simulink library "cstblocks"  (Simulink 7.4)
settings: Solver=ode45  SolverMode=SingleTasking  StartTime=0.0  StopTime=10.0  RelTol=1e-3
values from neighbouring files (symbols this model uses):
  D = diag(D)    [care.m]    (also in delayss.m = getPrivateData(sys); gcare.m = []; gdare.m = [])
libraries: cstextras x3
settings Model: RequirementInfo=9  ForwardingTableString=||__slOldName__||cstblocks/Output Point||__slNewName__||slctrlobsolete/Output Point||__slOldName__||cstblocks/Input Point||__slNewName__||slctrlobsolete/Input Point  Creator=greg  LastModifiedBy=pascal

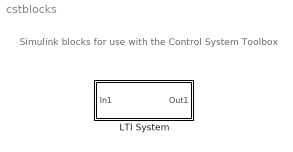
== system cstblocks ==
  note: Simulink blocks for use with the
      | Control System Toolbox
  LTI System : Subsystem  BlockChoice=CSS  mask(LTI Block){sys=tf(1,[1 1]), IC=[]}
      mask prompts: sys "LTI system variable"; IC "Initial states (state-space only)"
      mask help:
      | The LTI System block accepts both continuous and discrete LTI models as defined in the Control System Toolbox. Transfer function, state-space, and zero-pole-gain formats are all supported in this block.
      |
      | Note: Initial states are only meaningful for state-space systems.
      mask init:
      | try
      |    % read data to initialize mask variables
      |    [D,Ts,Tdi,Tdo,Tdio,x0,sysname]=...
      |       ltimask('Initialize',gcb,sys,IC);
      |    % update contents
      |    model = bdroot;
      |    df = get_param(model,'dirty');
      |    ltimask('UpdateDiagram',gcb,D,Ts,Tdio);
      |    try      
      |       % Attempt to modify locked library -> error
      |       % Makes block show ??? when loading CSTBLOCKS
      |       % for the first time
      |       set_param(model,'dirty',df)
      |    end
      | catch ME
      |    sys = [];  IC = [];   sysname = '???';
      |    throw(ME)
      | end
      mask Help:
      | The LTI System block accepts any of the three standard LTI models described in the Control System Toolbox: transfer function, zero/pole/gain, or state space. Internally, LTI models will be converted to their state space equivalent for evaluation.
      | <p>
      | In the editable text box labeled <b>LTI System Variable</b>, enter a valid LTI model.
      | <p>
      | In the editable text box labeled <b>Initial States</b> enter the initial state vector.  Initial states are only valid for state-space systems.
      | <p>
      | See also TF, ZPK, SS, LTIMODELS.
      mask CallbackString: ltimask('MaskLTICallback',gcb);|
      mask Display: disp(sysname)

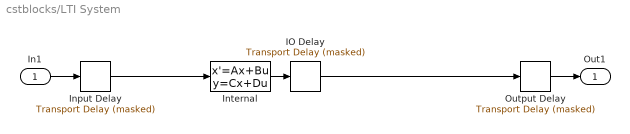
== system cstblocks/LTI System ==
  In1 : Inport  OutDataType=sfix(16)  OutScaling=2^0
  IO Delay : cstextras/Transport Delay (masked)  SystemSampleTime=-1  Td=Tdio  u0=0  bufsize=1024
  Input Delay : cstextras/Transport Delay (masked)  SystemSampleTime=-1  Td=Tdi  u0=0  bufsize=1024
  Internal : StateSpace  A=D.a  B=D.b  C=D.c  D=D.d
  Output Delay : cstextras/Transport Delay (masked)  SystemSampleTime=-1  Td=Tdo  u0=0  bufsize=1024
  Out1 : Outport  OutDataType=sfix(16)  OutScaling=2^0  InitialOutput=0
  wires:
  In1/1 -> Input Delay/1
  Output Delay/1 -> Out1/1
  Input Delay/1 -> Internal/1
  Internal/1 -> IO Delay/1
  IO Delay/1 -> Output Delay/1
